simulink model "lab4simulink2018"  (R2018a)
settings: Solver=VariableStepAuto  StartTime=0.0  StopTime=10.0  RelTol=1e-3
undefined symbols (not defined in the file): K_bes
settings Model: LastModifiedBy=clboland
settings DataIOCC: ReturnWorkspaceOutputs=on
settings DebuggingCC: UnconnectedInputMsg=none  UnconnectedOutputMsg=none  UnconnectedLineMsg=none
settings ModelReferenceCC: EnableRefExpFcnMdlSchedulingChecks=off
settings SFSimCC: SimUseLocalCustomCode=on
settings RTWCC: Description=Generic Real-Time Target  RTWUseLocalCustomCode=on

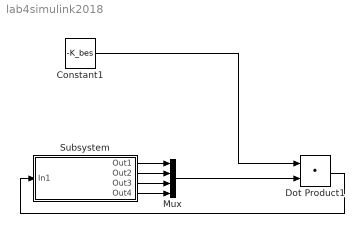
== system lab4simulink2018 ==
  Constant1 : Constant  Value=-K_bes
  Dot Product1 : DotProduct  InputSameDT=on  OutDataTypeStr=Inherit: Inherit via internal rule
  Mux : Mux
  Subsystem : Subsystem
  wires:
  Subsystem/1(Out1) -> Mux/1
  Subsystem/2(Out2) -> Mux/2
  Subsystem/3(Out3) -> Mux/3
  Subsystem/4(Out4) -> Mux/4
  Mux/1 -> Dot Product1/2
  Constant1/1 -> Dot Product1/1
  Dot Product1/1 -> Subsystem/1(In1)

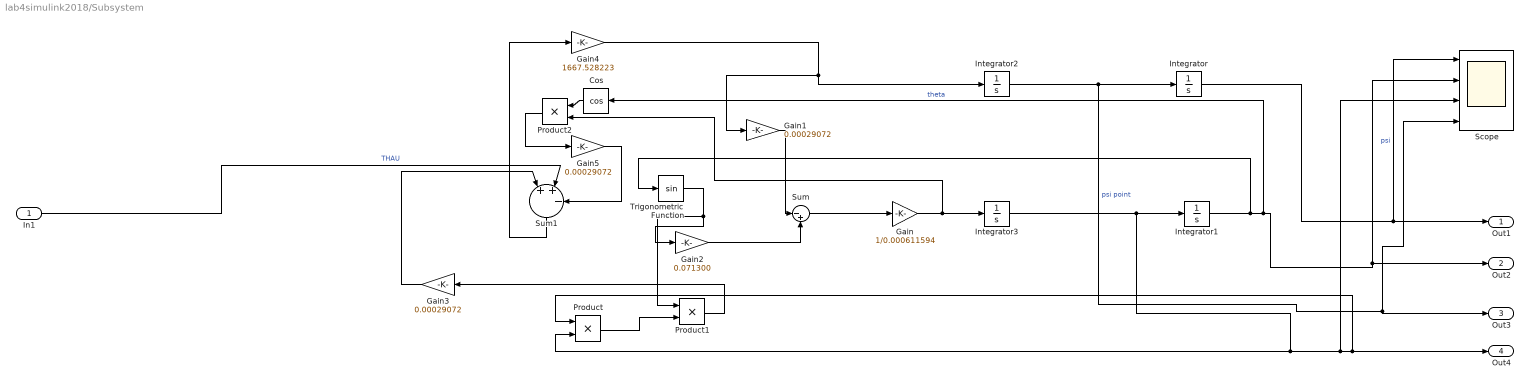
== system lab4simulink2018/Subsystem ==
  In1 : Inport
  Cos : Trigonometry  Operator=cos
  Gain : Gain  Gain=1/0.000611594
  Gain1 : Gain  Gain=0.00029072
  Gain2 : Gain  Gain=0.071300
  Gain3 : Gain  Gain=0.00029072
  Gain4 : Gain  Gain=1667.528223
  Gain5 : Gain  Gain=0.00029072
  Integrator : Integrator
  Integrator1 : Integrator  InitialCondition=deg2rad(10)
  Integrator2 : Integrator
  Integrator3 : Integrator
  Product : Product
  Product1 : Product
  Product2 : Product
  Scope : Scope  NumInputPorts=4
  Sum : Sum  Inputs=|-+
  Sum1 : Sum  Inputs=|++-
  Trigonometric Function : Trigonometry
  Out1 : Outport  VectorParamsAs1DForOutWhenUnconnected=on
  Out2 : Outport  Port=2  VectorParamsAs1DForOutWhenUnconnected=on
  Out3 : Outport  Port=3  VectorParamsAs1DForOutWhenUnconnected=on
  Out4 : Outport  Port=4  VectorParamsAs1DForOutWhenUnconnected=on
  wires:
  Integrator2/1 -> Out3/1, Scope/4, Integrator/1  "psi point"
  Sum/1 -> Gain/1
  Gain4/1 -> Integrator2/1, Gain1/1
  Gain1/1 -> Sum/1
  Gain2/1 -> Sum/2
  Integrator3/1 -> Product/2, Out4/1, Product/1, Scope/3, Integrator1/1
  Product/1 -> Product1/2
  Trigonometric Function/1 -> Product1/1, Gain2/1
  In1/1 -> Sum1/2  "THAU"
  Product1/1 -> Gain3/1
  Gain3/1 -> Sum1/1
  Sum1/1 -> Gain4/1
  Cos/1 -> Product2/1
  Gain/1 -> Product2/2, Integrator3/1
  Product2/1 -> Gain5/1
  Gain5/1 -> Sum1/3
  Integrator/1 -> Out1/1, Scope/1  "psi"
  Integrator1/1 -> Trigonometric Function/1, Cos/1, Out2/1, Scope/2  "theta"
